simulink model "microwave_class_updated"  (Simulink 8.5)
settings: Solver=FixedStepDiscrete  StartTime=0.0  StopTime=inf  MaxStep=1  RelTol=1e-3
libraries: microwave_class_defs x36, sldvlib x21, powerlib_meascontrol x13, simulink x9
settings Model: Creator=spmiller  LastModifiedBy=Elaheh
settings DataIOCC: SaveFormat=Structure
settings OptimizationCC: InitFltsAndDblsToZero=on
settings DebuggingCC: SaveWithParameterizedLinksMsg=none  SignalResolutionControl=TryResolveAllWithWarning  SolverPrmCheckMsg=warning  MultiTaskDSMMsg=warning  MultiTaskCondExecSysMsg=none  FcnCallInpInsideContextMsg=UseLocalSettings
settings SFSimCC: SimParseCustomCode=off
settings GRTTargetCC: TargetFcnLib=ansi_tfl_tmw.mat

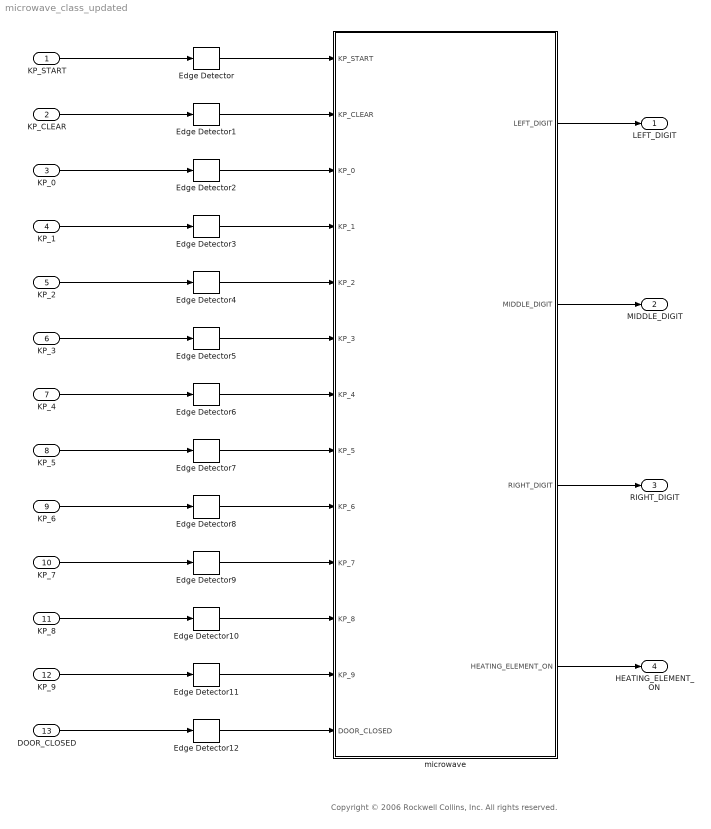
== system microwave_class_updated ==
  note: Copyright © 2006 Rockwell Collins, Inc. All rights reserved.
  KP_START : Inport  OutDataTypeStr=boolean
  KP_CLEAR : Inport  Port=2  OutDataTypeStr=boolean
  KP_0 : Inport  Port=3  OutDataTypeStr=boolean
  KP_1 : Inport  Port=4  OutDataTypeStr=boolean
  KP_2 : Inport  Port=5  OutDataTypeStr=boolean
  KP_3 : Inport  Port=6  OutDataTypeStr=boolean
  KP_4 : Inport  Port=7  OutDataTypeStr=boolean
  KP_5 : Inport  Port=8  OutDataTypeStr=boolean
  KP_6 : Inport  Port=9  OutDataTypeStr=boolean
  KP_7 : Inport  Port=10  OutDataTypeStr=boolean
  KP_8 : Inport  Port=11  OutDataTypeStr=boolean
  KP_9 : Inport  Port=12  OutDataTypeStr=boolean
  DOOR_CLOSED : Inport  Port=13  OutDataTypeStr=boolean
  Edge Detector{,1..12} (13 alike) : powerlib_meascontrol/Logic/Edge Detector  model=Rising  ic=0  Ts=0
  microwave : Subsystem
  LEFT_DIGIT : Outport  OutDataTypeStr=int8
  MIDDLE_DIGIT : Outport  Port=2  OutDataTypeStr=int8
  RIGHT_DIGIT : Outport  Port=3  OutDataTypeStr=int8
  HEATING_ELEMENT_ON : Outport  Port=4  OutDataTypeStr=boolean
  wires:
  KP_START/1 -> Edge Detector/1
  microwave/2(MIDDLE_DIGIT) -> MIDDLE_DIGIT/1
  microwave/3(RIGHT_DIGIT) -> RIGHT_DIGIT/1
  microwave/4(HEATING_ELEMENT_ON) -> HEATING_ELEMENT_ON/1
  microwave/1(LEFT_DIGIT) -> LEFT_DIGIT/1
  KP_3/1 -> Edge Detector5/1
  KP_4/1 -> Edge Detector6/1
  KP_6/1 -> Edge Detector8/1
  KP_7/1 -> Edge Detector9/1
  KP_9/1 -> Edge Detector11/1
  DOOR_CLOSED/1 -> Edge Detector12/1
  Edge Detector/1 -> microwave/1(KP_START)
  KP_CLEAR/1 -> Edge Detector1/1
  Edge Detector1/1 -> microwave/2(KP_CLEAR)
  KP_0/1 -> Edge Detector2/1
  Edge Detector2/1 -> microwave/3(KP_0)
  KP_1/1 -> Edge Detector3/1
  Edge Detector3/1 -> microwave/4(KP_1)
  KP_2/1 -> Edge Detector4/1
  Edge Detector4/1 -> microwave/5(KP_2)
  Edge Detector5/1 -> microwave/6(KP_3)
  Edge Detector6/1 -> microwave/7(KP_4)
  Edge Detector7/1 -> microwave/8(KP_5)
  KP_5/1 -> Edge Detector7/1
  Edge Detector8/1 -> microwave/9(KP_6)
  Edge Detector9/1 -> microwave/10(KP_7)
  Edge Detector10/1 -> microwave/11(KP_8)
  KP_8/1 -> Edge Detector10/1
  Edge Detector11/1 -> microwave/12(KP_9)
  Edge Detector12/1 -> microwave/13(DOOR_CLOSED)

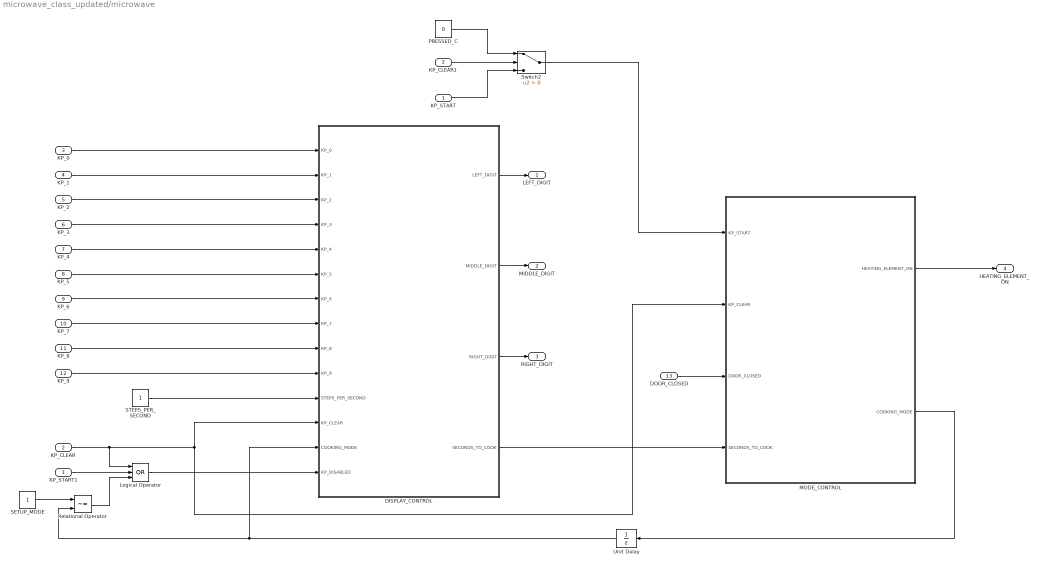
== system microwave_class_updated/microwave ==
  KP_START : Inport  OutDataTypeStr=boolean
  KP_CLEAR : Inport  Port=2  OutDataTypeStr=boolean
  KP_0 : Inport  Port=3  OutDataTypeStr=boolean
  KP_1 : Inport  Port=4  OutDataTypeStr=boolean
  KP_2 : Inport  Port=5  OutDataTypeStr=boolean
  KP_3 : Inport  Port=6  OutDataTypeStr=boolean
  KP_4 : Inport  Port=7  OutDataTypeStr=boolean
  KP_5 : Inport  Port=8  OutDataTypeStr=boolean
  KP_6 : Inport  Port=9  OutDataTypeStr=boolean
  KP_7 : Inport  Port=10  OutDataTypeStr=boolean
  KP_8 : Inport  Port=11  OutDataTypeStr=boolean
  KP_9 : Inport  Port=12  OutDataTypeStr=boolean
  DOOR_CLOSED : Inport  Port=13  OutDataTypeStr=boolean
  DISPLAY_CONTROL : Subsystem
  KP_CLEAR1 : InportShadow  Port=2  OutDataTypeStr=boolean
  KP_START1 : InportShadow  OutDataTypeStr=boolean
  Logical Operator : Logic  Operator=OR  Inputs=3  AllPortsSameDT=off  OutDataTypeStr=boolean
  MODE_CONTROL : Subsystem
  PRESSED_C : Constant  Value=0  OutDataTypeStr=boolean
  Relational Operator : RelationalOperator  Operator=~=  OutDataTypeStr=boolean
  SETUP_MODE : Constant  OutDataTypeStr=int8
  STEPS_PER_SECOND : Constant  OutDataTypeStr=int8
  Switch2 : Switch  Criteria=u2 > Threshold
  Unit Delay : UnitDelay  SampleTime=-1
  LEFT_DIGIT : Outport  OutDataTypeStr=int8
  MIDDLE_DIGIT : Outport  Port=2  OutDataTypeStr=int8
  RIGHT_DIGIT : Outport  Port=3  OutDataTypeStr=int8
  HEATING_ELEMENT_ON : Outport  Port=4  OutDataTypeStr=boolean
  wires:
  KP_CLEAR/1 -> Logical Operator/1, DISPLAY_CONTROL/12(KP_CLEAR), MODE_CONTROL/2(KP_CLEAR)
  DISPLAY_CONTROL/4(SECONDS_TO_COOK) -> MODE_CONTROL/4(SECONDS_TO_COOK)
  MODE_CONTROL/2(COOKING_MODE) -> Unit Delay/1
  Unit Delay/1 -> Relational Operator/2, DISPLAY_CONTROL/13(COOKING_MODE)
  DOOR_CLOSED/1 -> MODE_CONTROL/3(DOOR_CLOSED)
  DISPLAY_CONTROL/3(RIGHT_DIGIT) -> RIGHT_DIGIT/1
  DISPLAY_CONTROL/2(MIDDLE_DIGIT) -> MIDDLE_DIGIT/1
  DISPLAY_CONTROL/1(LEFT_DIGIT) -> LEFT_DIGIT/1
  MODE_CONTROL/1(HEATING_ELEMENT_ON) -> HEATING_ELEMENT_ON/1
  STEPS_PER_SECOND/1 -> DISPLAY_CONTROL/11(STEPS_PER_SECOND)
  KP_CLEAR1/1 -> Switch2/2
  PRESSED_C/1 -> Switch2/1
  KP_START/1 -> Switch2/3
  KP_1/1 -> DISPLAY_CONTROL/2(KP_1)
  KP_3/1 -> DISPLAY_CONTROL/4(KP_3)
  KP_4/1 -> DISPLAY_CONTROL/5(KP_4)
  KP_5/1 -> DISPLAY_CONTROL/6(KP_5)
  KP_6/1 -> DISPLAY_CONTROL/7(KP_6)
  KP_7/1 -> DISPLAY_CONTROL/8(KP_7)
  KP_2/1 -> DISPLAY_CONTROL/3(KP_2)
  KP_8/1 -> DISPLAY_CONTROL/9(KP_8)
  KP_9/1 -> DISPLAY_CONTROL/10(KP_9)
  KP_0/1 -> DISPLAY_CONTROL/1(KP_0)
  KP_START1/1 -> Logical Operator/2
  Logical Operator/1 -> DISPLAY_CONTROL/14(KP_DISABLED)
  Relational Operator/1 -> Logical Operator/3
  SETUP_MODE/1 -> Relational Operator/1
  Switch2/1 -> MODE_CONTROL/1(KP_START)

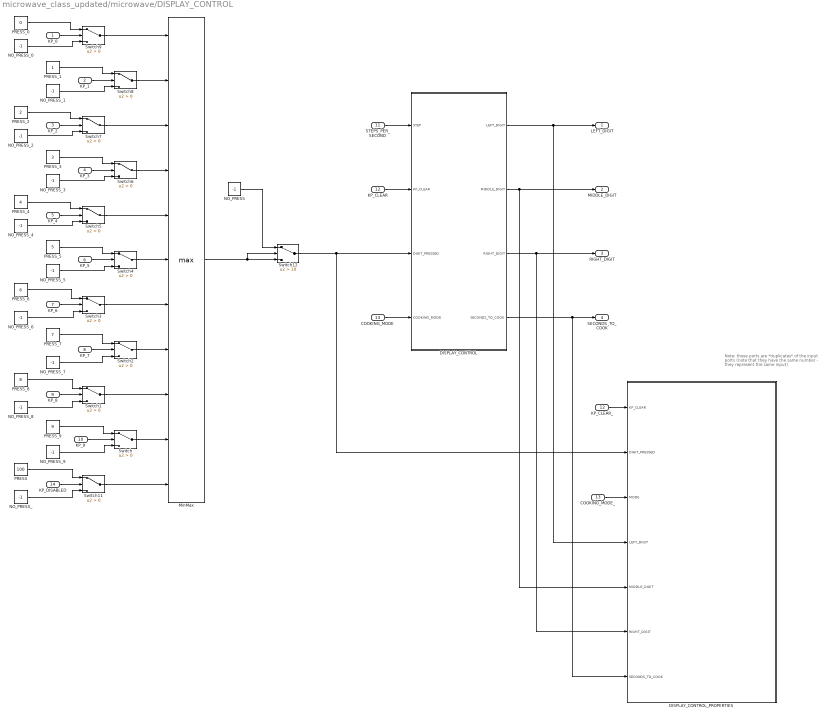
== system microwave_class_updated/microwave/DISPLAY_CONTROL ==
  note: Note: these ports are *duplicates* of the
      | input ports (note that they have the same
      | number - they represent the same input)
  KP_0 : Inport
  KP_1 : Inport  Port=2
  KP_2 : Inport  Port=3
  KP_3 : Inport  Port=4
  KP_4 : Inport  Port=5
  KP_5 : Inport  Port=6
  KP_6 : Inport  Port=7
  KP_7 : Inport  Port=8
  KP_8 : Inport  Port=9
  KP_9 : Inport  Port=10
  STEPS_PER_SECOND : Inport  Port=11  OutDataTypeStr=int8
  KP_CLEAR : Inport  Port=12
  COOKING_MODE : Inport  Port=13  OutDataTypeStr=uint8
  KP_DISABLED : Inport  Port=14
  COOKING_MODE_ : InportShadow  Port=13  OutDataTypeStr=uint8
  DISPLAY_CONTROL : Stateflow chart  TreatAsAtomicUnit=on
  DISPLAY_CONTROL_PROPERTIES : Subsystem
  KP_CLEAR_ : InportShadow  Port=12
  MinMax : MinMax  Function=max  Inputs=11
  NO_PRESS : Constant  Value=-1  OutDataTypeStr=int8
  NO_PRESS_{,0..9} (11 alike) : Constant  Value=-1  OutDataTypeStr=int8
  PRESS : Constant  Value=100  OutDataTypeStr=int8
  PRESS_0 : Constant  Value=0  OutDataTypeStr=int8
  PRESS_1 : Constant  OutDataTypeStr=int8
  PRESS_2 : Constant  Value=2  OutDataTypeStr=int8
  PRESS_3 : Constant  Value=3  OutDataTypeStr=int8
  PRESS_4 : Constant  Value=4  OutDataTypeStr=int8
  PRESS_5 : Constant  Value=5  OutDataTypeStr=int8
  PRESS_6 : Constant  Value=6  OutDataTypeStr=int8
  PRESS_7 : Constant  Value=7  OutDataTypeStr=int8
  PRESS_8 : Constant  Value=8  OutDataTypeStr=int8
  PRESS_9 : Constant  Value=9  OutDataTypeStr=int8
  Switch{,1..9,11} (11 alike) : Switch  Criteria=u2 > Threshold
  Switch12 : Switch  Criteria=u2 > Threshold  Threshold=10
  LEFT_DIGIT : Outport  OutDataTypeStr=int8
  MIDDLE_DIGIT : Outport  Port=2  OutDataTypeStr=int8
  RIGHT_DIGIT : Outport  Port=3  OutDataTypeStr=int8
  SECONDS_TO_COOK : Outport  Port=4  OutDataTypeStr=int8
  wires:
  STEPS_PER_SECOND/1 -> DISPLAY_CONTROL/1(STEP)
  DISPLAY_CONTROL/1(LEFT_DIGIT) -> DISPLAY_CONTROL_PROPERTIES/4(LEFT_DIGIT), LEFT_DIGIT/1
  DISPLAY_CONTROL/3(RIGHT_DIGIT) -> RIGHT_DIGIT/1, DISPLAY_CONTROL_PROPERTIES/6(RIGHT_DIGIT)
  DISPLAY_CONTROL/2(MIDDLE_DIGIT) -> DISPLAY_CONTROL_PROPERTIES/5(MIDDLE_DIGIT), MIDDLE_DIGIT/1
  KP_CLEAR/1 -> DISPLAY_CONTROL/2(KP_CLEAR)
  NO_PRESS_9/1 -> Switch/3
  KP_9/1 -> Switch/2
  PRESS_9/1 -> Switch/1
  PRESS_8/1 -> Switch1/1
  NO_PRESS_8/1 -> Switch1/3
  KP_8/1 -> Switch1/2
  KP_7/1 -> Switch2/2
  PRESS_7/1 -> Switch2/1
  NO_PRESS_7/1 -> Switch2/3
  KP_6/1 -> Switch3/2
  PRESS_6/1 -> Switch3/1
  NO_PRESS_6/1 -> Switch3/3
  KP_5/1 -> Switch4/2
  PRESS_5/1 -> Switch4/1
  NO_PRESS_5/1 -> Switch4/3
  PRESS_4/1 -> Switch5/1
  NO_PRESS_4/1 -> Switch5/3
  KP_4/1 -> Switch5/2
  KP_3/1 -> Switch6/2
  PRESS_3/1 -> Switch6/1
  NO_PRESS_3/1 -> Switch6/3
  PRESS_2/1 -> Switch7/1
  NO_PRESS_2/1 -> Switch7/3
  KP_2/1 -> Switch7/2
  KP_1/1 -> Switch8/2
  PRESS_1/1 -> Switch8/1
  NO_PRESS_1/1 -> Switch8/3
  PRESS_0/1 -> Switch9/1
  NO_PRESS_0/1 -> Switch9/3
  KP_0/1 -> Switch9/2
  Switch2/1 -> MinMax/8
  Switch1/1 -> MinMax/9
  Switch/1 -> MinMax/10
  COOKING_MODE_/1 -> DISPLAY_CONTROL_PROPERTIES/3(MODE)
  KP_CLEAR_/1 -> DISPLAY_CONTROL_PROPERTIES/1(KP_CLEAR)
  COOKING_MODE/1 -> DISPLAY_CONTROL/4(COOKING_MODE)
  DISPLAY_CONTROL/4(SECONDS_TO_COOK) -> DISPLAY_CONTROL_PROPERTIES/7(SECONDS_TO_COOK), SECONDS_TO_COOK/1
  Switch3/1 -> MinMax/7
  Switch4/1 -> MinMax/6
  Switch5/1 -> MinMax/5
  Switch6/1 -> MinMax/4
  Switch7/1 -> MinMax/3
  Switch8/1 -> MinMax/2
  Switch9/1 -> MinMax/1
  Switch12/1 -> DISPLAY_CONTROL_PROPERTIES/2(DIGIT_PRESSED), DISPLAY_CONTROL/3(DIGIT_PRESSED)
  NO_PRESS/1 -> Switch12/1
  PRESS/1 -> Switch11/1
  NO_PRESS_/1 -> Switch11/3
  KP_DISABLED/1 -> Switch11/2
  Switch11/1 -> MinMax/11
  MinMax/1 -> Switch12/2, Switch12/3

== system microwave_class_updated/microwave/MODE_CONTROL ==
  KP_START : Inport  OutDataTypeStr=boolean
  KP_CLEAR : Inport  Port=2  OutDataTypeStr=boolean
  DOOR_CLOSED : Inport  Port=3  OutDataTypeStr=boolean
  SECONDS_TO_COOK : Inport  Port=4
  MODE_CONTROL : Stateflow chart  TreatAsAtomicUnit=on
  MODE_CONTROL_PROPERTIES : Subsystem
  HEATING_ELEMENT_ON : Outport
  COOKING_MODE : Outport  Port=2
  wires:
  KP_START/1 -> MODE_CONTROL_PROPERTIES/1(KP_START), MODE_CONTROL/1(KP_START)
  KP_CLEAR/1 -> MODE_CONTROL_PROPERTIES/2(KP_CLEAR), MODE_CONTROL/2(KP_CLEAR)
  DOOR_CLOSED/1 -> MODE_CONTROL_PROPERTIES/3(DOOR_CLOSED), MODE_CONTROL/3(DOOR_CLOSED)
  SECONDS_TO_COOK/1 -> MODE_CONTROL_PROPERTIES/4(SECONDS_TO_COOK), MODE_CONTROL/4(SECONDS_TO_COOK)
  MODE_CONTROL/1(COOKING_MODE) -> MODE_CONTROL_PROPERTIES/5(COOKING_MODE), COOKING_MODE/1
  MODE_CONTROL/2(HEATING_ELEMENT_ON) -> MODE_CONTROL_PROPERTIES/6(HEATING_ELEMENT_ON), HEATING_ELEMENT_ON/1

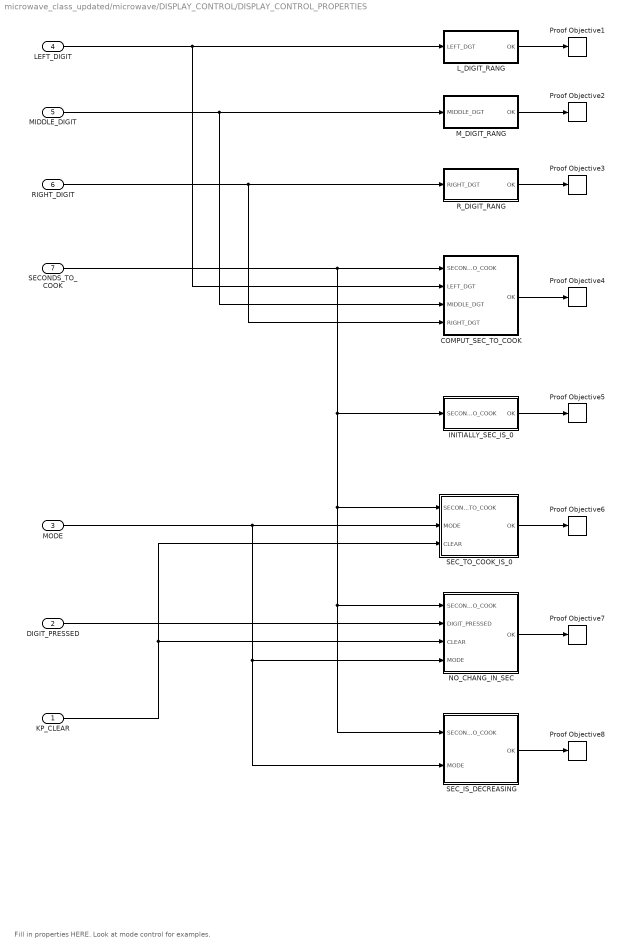
== system microwave_class_updated/microwave/DISPLAY_CONTROL/DISPLAY_CONTROL_PROPERTIES ==
  note: Fill in properties HERE. Look at mode control for examples.
  KP_CLEAR : Inport  OutDataTypeStr=boolean
  DIGIT_PRESSED : Inport  Port=2  OutDataTypeStr=int8
  MODE : Inport  Port=3  OutDataTypeStr=uint8
  LEFT_DIGIT : Inport  Port=4  OutDataTypeStr=int8
  MIDDLE_DIGIT : Inport  Port=5  OutDataTypeStr=int8
  RIGHT_DIGIT : Inport  Port=6  OutDataTypeStr=int8
  SECONDS_TO_COOK : Inport  Port=7
  COMPUT_SEC_TO_COOK : Subsystem
  INITIALLY_SEC_IS_0 : Subsystem
  L_DIGIT_RANG : Subsystem
  M_DIGIT_RANG : Subsystem
  NO_CHANG_IN_SEC : Subsystem
  Proof Objective{1..8} (8 alike) : sldvlib/Objectives and Constraints/Proof Objective  enabled=on  customAVTBlockType=Proof Objective  intervals=true  dispValues=on  outEnabled=on  enableStopSim=off
      settings: AttributesFormatString=%<intervals>
  R_DIGIT_RANG : Subsystem
  SEC_IS_DECREASING : Subsystem
  SEC_TO_COOK_IS_0 : Subsystem
  wires:
  L_DIGIT_RANG/1(OK) -> Proof Objective1/1
  M_DIGIT_RANG/1(OK) -> Proof Objective2/1
  R_DIGIT_RANG/1(OK) -> Proof Objective3/1
  COMPUT_SEC_TO_COOK/1(OK) -> Proof Objective4/1
  INITIALLY_SEC_IS_0/1(OK) -> Proof Objective5/1
  SEC_TO_COOK_IS_0/1(OK) -> Proof Objective6/1
  NO_CHANG_IN_SEC/1(OK) -> Proof Objective7/1
  SEC_IS_DECREASING/1(OK) -> Proof Objective8/1
  MODE/1 -> SEC_IS_DECREASING/2(MODE), NO_CHANG_IN_SEC/4(MODE), SEC_TO_COOK_IS_0/2(MODE)
  LEFT_DIGIT/1 -> COMPUT_SEC_TO_COOK/2(LEFT_DGT), L_DIGIT_RANG/1(LEFT_DGT)
  MIDDLE_DIGIT/1 -> COMPUT_SEC_TO_COOK/3(MIDDLE_DGT), M_DIGIT_RANG/1(MIDDLE_DGT)
  SECONDS_TO_COOK/1 -> SEC_IS_DECREASING/1(SECONDS_TO_COOK), NO_CHANG_IN_SEC/1(SECONDS_TO_COOK), SEC_TO_COOK_IS_0/1(SECONDS_TO_COOK), INITIALLY_SEC_IS_0/1(SECONDS_TO_COOK), COMPUT_SEC_TO_COOK/1(SECONDS_TO_COOK)
  DIGIT_PRESSED/1 -> NO_CHANG_IN_SEC/2(DIGIT_PRESSED)
  KP_CLEAR/1 -> SEC_TO_COOK_IS_0/3(CLEAR), NO_CHANG_IN_SEC/3(CLEAR)
  RIGHT_DIGIT/1 -> COMPUT_SEC_TO_COOK/4(RIGHT_DGT), R_DIGIT_RANG/1(RIGHT_DGT)

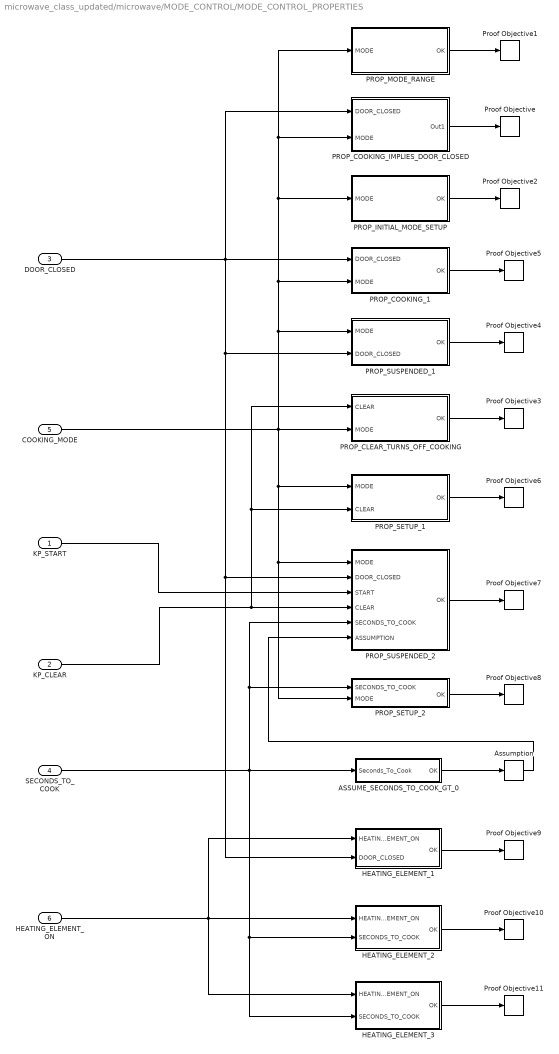
== system microwave_class_updated/microwave/MODE_CONTROL/MODE_CONTROL_PROPERTIES ==
  KP_START : Inport  OutDataTypeStr=boolean
  KP_CLEAR : Inport  Port=2  OutDataTypeStr=boolean
  DOOR_CLOSED : Inport  Port=3  OutDataTypeStr=boolean
  SECONDS_TO_COOK : Inport  Port=4
  COOKING_MODE : Inport  Port=5  OutDataTypeStr=uint8
  HEATING_ELEMENT_ON : Inport  Port=6  OutDataTypeStr=boolean
  ASSUME_SECONDS_TO_COOK_GT_0 : Subsystem
  Assumption : sldvlib/Objectives and Constraints/Assumption  enabled=on  customAVTBlockType=Assumption  intervals=true  initial=off  dispValues=on  outEnabled=on
      settings: AttributesFormatString=%<intervals>
  HEATING_ELEMENT_1 : Subsystem
  HEATING_ELEMENT_2 : Subsystem
  HEATING_ELEMENT_3 : Subsystem
  PROP_CLEAR_TURNS_OFF_COOKING : Subsystem
  PROP_COOKING_1 : Subsystem
  PROP_COOKING_IMPLIES_DOOR_CLOSED : Subsystem
  PROP_INITIAL_MODE_SETUP : Subsystem
  PROP_MODE_RANGE : Subsystem
  PROP_SETUP_1 : Subsystem
  PROP_SETUP_2 : Subsystem
  PROP_SUSPENDED_1 : Subsystem
  PROP_SUSPENDED_2 : Subsystem
  Proof Objective{,1..11} (12 alike) : sldvlib/Objectives and Constraints/Proof Objective  enabled=on  customAVTBlockType=Proof Objective  intervals=true  dispValues=on  outEnabled=on  enableStopSim=off
      settings: AttributesFormatString=%<intervals>
  wires:
  COOKING_MODE/1 -> PROP_SUSPENDED_1/1(MODE), PROP_INITIAL_MODE_SETUP/1(MODE), PROP_MODE_RANGE/1(MODE), PROP_COOKING_IMPLIES_DOOR_CLOSED/2(MODE), PROP_COOKING_1/2(MODE), PROP_SETUP_2/2(MODE), PROP_SUSPENDED_2/1(MODE), PROP_SETUP_1/1(MODE), PROP_CLEAR_TURNS_OFF_COOKING/2(MODE)
  PROP_COOKING_IMPLIES_DOOR_CLOSED/1(Out1) -> Proof Objective/1
  PROP_CLEAR_TURNS_OFF_COOKING/1(OK) -> Proof Objective3/1
  ASSUME_SECONDS_TO_COOK_GT_0/1(OK) -> Assumption/1
  PROP_MODE_RANGE/1(OK) -> Proof Objective1/1
  PROP_INITIAL_MODE_SETUP/1(OK) -> Proof Objective2/1
  PROP_SUSPENDED_1/1(OK) -> Proof Objective4/1
  PROP_COOKING_1/1(OK) -> Proof Objective5/1
  PROP_SETUP_1/1(OK) -> Proof Objective6/1
  PROP_SUSPENDED_2/1(OK) -> Proof Objective7/1
  PROP_SETUP_2/1(OK) -> Proof Objective8/1
  KP_CLEAR/1 -> PROP_CLEAR_TURNS_OFF_COOKING/1(CLEAR), PROP_SETUP_1/2(CLEAR), PROP_SUSPENDED_2/4(CLEAR)
  DOOR_CLOSED/1 -> PROP_COOKING_IMPLIES_DOOR_CLOSED/1(DOOR_CLOSED), HEATING_ELEMENT_1/2(DOOR_CLOSED), PROP_SUSPENDED_2/2(DOOR_CLOSED), PROP_SUSPENDED_1/2(DOOR_CLOSED), PROP_COOKING_1/1(DOOR_CLOSED)
  KP_START/1 -> PROP_SUSPENDED_2/3(START)
  SECONDS_TO_COOK/1 -> HEATING_ELEMENT_2/2(SECONDS_TO_COOK), HEATING_ELEMENT_3/2(SECONDS_TO_COOK), PROP_SUSPENDED_2/5(SECONDS_TO_COOK), PROP_SETUP_2/1(SECONDS_TO_COOK), ASSUME_SECONDS_TO_COOK_GT_0/1(Seconds_To_Cook)
  HEATING_ELEMENT_1/1(OK) -> Proof Objective9/1
  HEATING_ELEMENT_2/1(OK) -> Proof Objective10/1
  HEATING_ELEMENT_3/1(OK) -> Proof Objective11/1
  HEATING_ELEMENT_ON/1 -> HEATING_ELEMENT_1/1(HEATING_ELEMENT_ON), HEATING_ELEMENT_3/1(HEATING_ELEMENT_ON), HEATING_ELEMENT_2/1(HEATING_ELEMENT_ON)
  Assumption/1 -> PROP_SUSPENDED_2/6(ASSUMPTION)

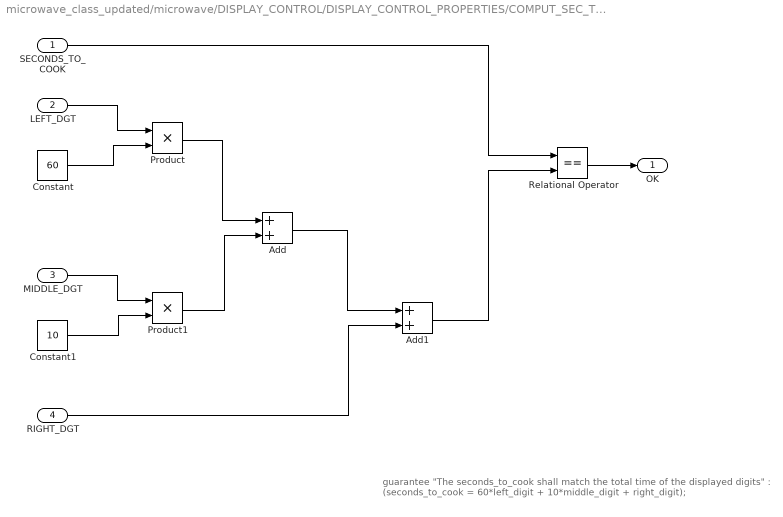
== system microwave_class_updated/microwave/DISPLAY_CONTROL/DISPLAY_CONTROL_PROPERTIES/COMPUT_SEC_TO_COOK ==
  note: guarantee "The seconds_to_cook shall match the total time of the displayed digits" :
      | 			(seconds_to_cook = 60*left_digit + 10*middle_digit + right_digit);
  SECONDS_TO_COOK : Inport
  LEFT_DGT : Inport  Port=2
  MIDDLE_DGT : Inport  Port=3
  RIGHT_DGT : Inport  Port=4
  Add : Sum
  Add1 : Sum
  Constant : Constant  Value=60
  Constant1 : Constant  Value=10
  Product : Product
  Product1 : Product
  Relational Operator : RelationalOperator  Operator===  OutDataTypeStr=boolean
  OK : Outport
  wires:
  SECONDS_TO_COOK/1 -> Relational Operator/1
  Relational Operator/1 -> OK/1
  LEFT_DGT/1 -> Product/1
  Constant/1 -> Product/2
  Product/1 -> Add/1
  MIDDLE_DGT/1 -> Product1/1
  Constant1/1 -> Product1/2
  Product1/1 -> Add/2
  RIGHT_DGT/1 -> Add1/2
  Add/1 -> Add1/1
  Add1/1 -> Relational Operator/2

== system microwave_class_updated/microwave/DISPLAY_CONTROL/DISPLAY_CONTROL_PROPERTIES/INITIALLY_SEC_IS_0 ==
  note: guarantee "Seconds to cook shall be initially zero" :
      | 			std.Initially(seconds_to_cook = 0);
  SECONDS_TO_COOK : Inport
  Constant : Constant  Value=0
  Relational Operator : RelationalOperator  Operator===  OutDataTypeStr=boolean
  initially_true : microwave_class_defs/initially_true
  OK : Outport
  wires:
  SECONDS_TO_COOK/1 -> Relational Operator/1
  Constant/1 -> Relational Operator/2
  Relational Operator/1 -> initially_true/1
  initially_true/1 -> OK/1

== system microwave_class_updated/microwave/DISPLAY_CONTROL/DISPLAY_CONTROL_PROPERTIES/L_DIGIT_RANG ==
  note: guarantee "left_digit range shall be [0..9]" :
      | 			(left_digit >= 0 and left_digit <= 9);
  LEFT_DGT : Inport
  Compare To Zero : simulink/Logic and Bit Operations/Compare To Zero  relop=>=  OutDataTypeStr=boolean
  Constant1 : Constant  Value=9
  Logical Operator : Logic  AllPortsSameDT=off  OutDataTypeStr=boolean
  Relational Operator : RelationalOperator  Operator=<=  OutDataTypeStr=boolean
  OK : Outport
  wires:
  LEFT_DGT/1 -> Compare To Zero/1, Relational Operator/1
  Constant1/1 -> Relational Operator/2
  Compare To Zero/1 -> Logical Operator/1
  Relational Operator/1 -> Logical Operator/2
  Logical Operator/1 -> OK/1

== system microwave_class_updated/microwave/DISPLAY_CONTROL/DISPLAY_CONTROL_PROPERTIES/M_DIGIT_RANG ==
  note: guarantee "middle_digit range shall be [0..9]" :
      | 			(middle_digit >= 0 and middle_digit <= 9);
  MIDDLE_DGT : Inport
  Compare To Zero : simulink/Logic and Bit Operations/Compare To Zero  relop=>=  OutDataTypeStr=boolean
  Constant1 : Constant  Value=9
  Logical Operator : Logic  AllPortsSameDT=off  OutDataTypeStr=boolean
  Relational Operator : RelationalOperator  Operator=<=  OutDataTypeStr=boolean
  OK : Outport
  wires:
  MIDDLE_DGT/1 -> Compare To Zero/1, Relational Operator/1
  Constant1/1 -> Relational Operator/2
  Compare To Zero/1 -> Logical Operator/1
  Relational Operator/1 -> Logical Operator/2
  Logical Operator/1 -> OK/1

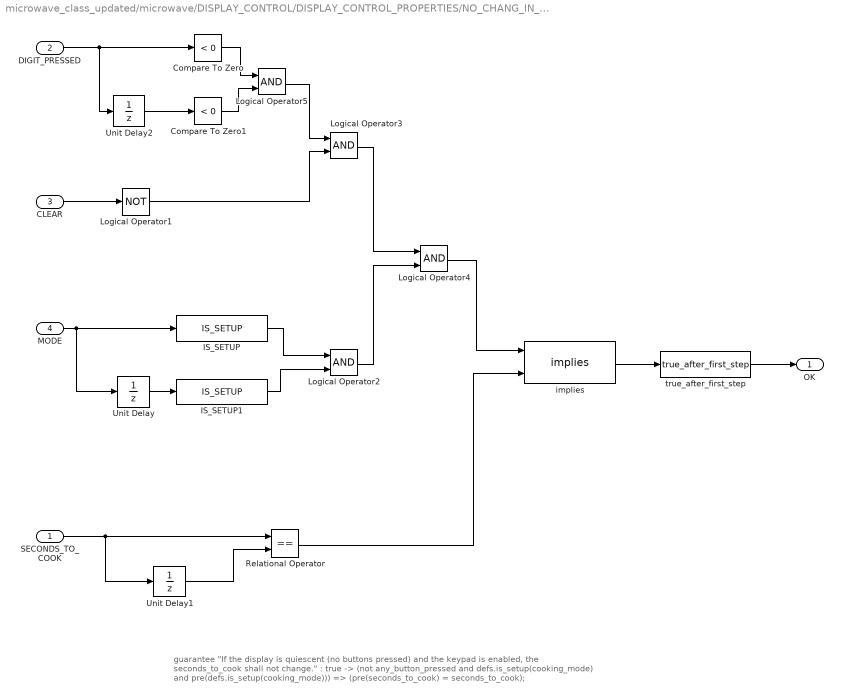
== system microwave_class_updated/microwave/DISPLAY_CONTROL/DISPLAY_CONTROL_PROPERTIES/NO_CHANG_IN_SEC ==
  note: guarantee "If the display is quiescent (no buttons pressed) and the keypad is enabled, the seconds_to_cook shall not change." :
      | 			true -> (not any_button_pressed and defs.is_setup(cooking_mode) and pre(defs.is_setup(cooking_mode))) => (pre(seconds_to_cook) = seconds_to_cook);
  SECONDS_TO_COOK : Inport
  DIGIT_PRESSED : Inport  Port=2
  CLEAR : Inport  Port=3
  MODE : Inport  Port=4
  Compare To Zero : simulink/Logic and Bit Operations/Compare To Zero  relop=<  OutDataTypeStr=boolean
  Compare To Zero1 : simulink/Logic and Bit Operations/Compare To Zero  relop=<  OutDataTypeStr=boolean
  IS_SETUP : microwave_class_defs/IS_SETUP
  IS_SETUP1 : microwave_class_defs/IS_SETUP
  Logical Operator1 : Logic  Operator=NOT  AllPortsSameDT=off  OutDataTypeStr=boolean
  Logical Operator{2..5} (4 alike) : Logic  AllPortsSameDT=off  OutDataTypeStr=boolean
  Relational Operator : RelationalOperator  Operator===  OutDataTypeStr=boolean
  Unit Delay : UnitDelay  SampleTime=-1
  Unit Delay1 : UnitDelay  SampleTime=-1
  Unit Delay2 : UnitDelay  SampleTime=-1
  implies : microwave_class_defs/implies
  true_after_first_step : microwave_class_defs/true_after_first_step
  OK : Outport
  wires:
  Logical Operator1/1 -> Logical Operator3/2
  Logical Operator3/1 -> Logical Operator4/1
  Relational Operator/1 -> implies/2
  implies/1 -> true_after_first_step/1
  true_after_first_step/1 -> OK/1
  CLEAR/1 -> Logical Operator1/1
  MODE/1 -> Unit Delay/1, IS_SETUP/1
  Unit Delay/1 -> IS_SETUP1/1
  IS_SETUP1/1 -> Logical Operator2/2
  IS_SETUP/1 -> Logical Operator2/1
  Logical Operator2/1 -> Logical Operator4/2
  Logical Operator4/1 -> implies/1
  SECONDS_TO_COOK/1 -> Unit Delay1/1, Relational Operator/1
  Unit Delay1/1 -> Relational Operator/2
  DIGIT_PRESSED/1 -> Unit Delay2/1, Compare To Zero/1
  Unit Delay2/1 -> Compare To Zero1/1
  Compare To Zero/1 -> Logical Operator5/1
  Compare To Zero1/1 -> Logical Operator5/2
  Logical Operator5/1 -> Logical Operator3/1

== system microwave_class_updated/microwave/DISPLAY_CONTROL/DISPLAY_CONTROL_PROPERTIES/R_DIGIT_RANG ==
  note: guarantee "right_digit range shall be [0..9]" :
      | 			(right_digit >= 0 and right_digit <= 9);
  RIGHT_DGT : Inport
  Compare To Zero : simulink/Logic and Bit Operations/Compare To Zero  relop=>=  OutDataTypeStr=boolean
  Constant1 : Constant  Value=9
  Logical Operator : Logic  AllPortsSameDT=off  OutDataTypeStr=boolean
  Relational Operator : RelationalOperator  Operator=<=  OutDataTypeStr=boolean
  OK : Outport
  wires:
  RIGHT_DGT/1 -> Compare To Zero/1, Relational Operator/1
  Constant1/1 -> Relational Operator/2
  Compare To Zero/1 -> Logical Operator/1
  Relational Operator/1 -> Logical Operator/2
  Logical Operator/1 -> OK/1

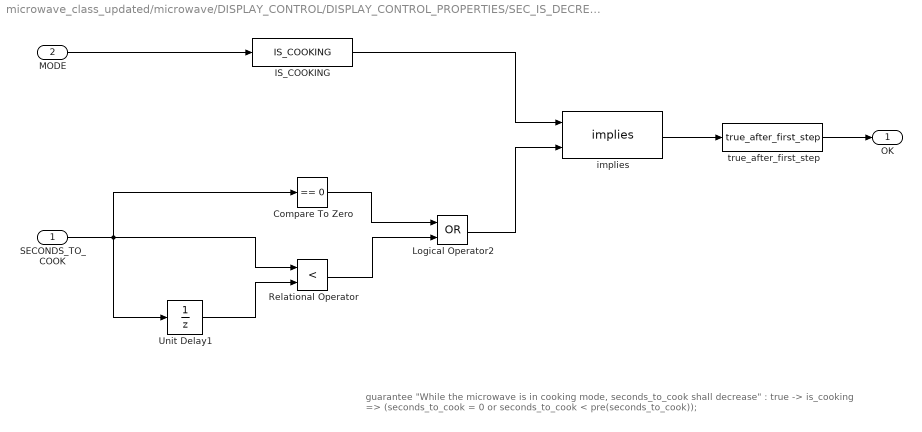
== system microwave_class_updated/microwave/DISPLAY_CONTROL/DISPLAY_CONTROL_PROPERTIES/SEC_IS_DECREASING ==
  note: guarantee "While the microwave is in cooking mode, seconds_to_cook shall decrease" :
      | 			true -> is_cooking => (seconds_to_cook = 0 or seconds_to_cook < pre(seconds_to_cook));
  SECONDS_TO_COOK : Inport
  MODE : Inport  Port=2
  Compare To Zero : simulink/Logic and Bit Operations/Compare To Zero  relop===  OutDataTypeStr=boolean
  IS_COOKING : microwave_class_defs/IS_COOKING
  Logical Operator2 : Logic  Operator=OR  AllPortsSameDT=off  OutDataTypeStr=boolean
  Relational Operator : RelationalOperator  Operator=<  OutDataTypeStr=boolean
  Unit Delay1 : UnitDelay  SampleTime=-1
  implies : microwave_class_defs/implies
  true_after_first_step : microwave_class_defs/true_after_first_step
  OK : Outport
  wires:
  Relational Operator/1 -> Logical Operator2/2
  implies/1 -> true_after_first_step/1
  true_after_first_step/1 -> OK/1
  MODE/1 -> IS_COOKING/1
  Logical Operator2/1 -> implies/2
  SECONDS_TO_COOK/1 -> Unit Delay1/1, Relational Operator/1, Compare To Zero/1
  Unit Delay1/1 -> Relational Operator/2
  Compare To Zero/1 -> Logical Operator2/1
  IS_COOKING/1 -> implies/1

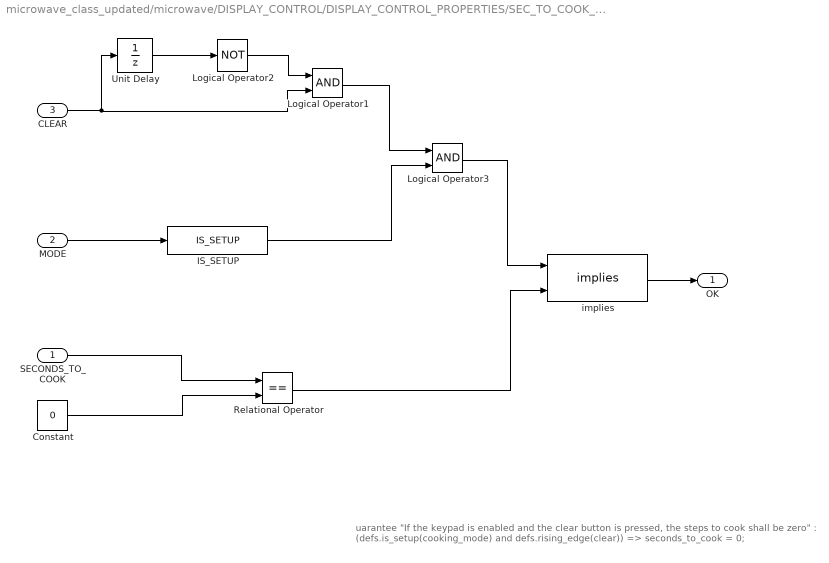
== system microwave_class_updated/microwave/DISPLAY_CONTROL/DISPLAY_CONTROL_PROPERTIES/SEC_TO_COOK_IS_0 ==
  note: uarantee "If the keypad is enabled and the clear button is pressed, the steps to cook shall be zero" :
      | 			(defs.is_setup(cooking_mode) and  defs.rising_edge(clear)) => seconds_to_cook = 0;
  SECONDS_TO_COOK : Inport
  MODE : Inport  Port=2
  CLEAR : Inport  Port=3
  Constant : Constant  Value=0
  IS_SETUP : microwave_class_defs/IS_SETUP
  Logical Operator1 : Logic  AllPortsSameDT=off  OutDataTypeStr=boolean
  Logical Operator2 : Logic  Operator=NOT  AllPortsSameDT=off  OutDataTypeStr=boolean
  Logical Operator3 : Logic  AllPortsSameDT=off  OutDataTypeStr=boolean
  Relational Operator : RelationalOperator  Operator===  OutDataTypeStr=boolean
  Unit Delay : UnitDelay  SampleTime=-1
  implies : microwave_class_defs/implies
  OK : Outport
  wires:
  SECONDS_TO_COOK/1 -> Relational Operator/1
  Constant/1 -> Relational Operator/2
  Unit Delay/1 -> Logical Operator2/1
  Logical Operator2/1 -> Logical Operator1/1
  CLEAR/1 -> Unit Delay/1, Logical Operator1/2
  Logical Operator1/1 -> Logical Operator3/1
  MODE/1 -> IS_SETUP/1
  IS_SETUP/1 -> Logical Operator3/2
  Logical Operator3/1 -> implies/1
  Relational Operator/1 -> implies/2
  implies/1 -> OK/1

== system microwave_class_updated/microwave/MODE_CONTROL/MODE_CONTROL_PROPERTIES/ASSUME_SECONDS_TO_COOK_GT_0 ==
  Seconds_To_Cook : Inport
  Constant : Constant  Value=0
  Relational Operator : RelationalOperator  OutDataTypeStr=boolean
  OK : Outport
  wires:
  Seconds_To_Cook/1 -> Relational Operator/1
  Constant/1 -> Relational Operator/2
  Relational Operator/1 -> OK/1

== system microwave_class_updated/microwave/MODE_CONTROL/MODE_CONTROL_PROPERTIES/HEATING_ELEMENT_1 ==
  note: guarantee "heating_element_on implies door_closed_sensor" :
      | 			heating_element_on => door_closed;
  HEATING_ELEMENT_ON : Inport
  DOOR_CLOSED : Inport  Port=2
  implies : microwave_class_defs/implies
  OK : Outport
  wires:
  HEATING_ELEMENT_ON/1 -> implies/1
  implies/1 -> OK/1
  DOOR_CLOSED/1 -> implies/2

== system microwave_class_updated/microwave/MODE_CONTROL/MODE_CONTROL_PROPERTIES/HEATING_ELEMENT_2 ==
  note: guarantee "heating element on implies time to cook decreases" :
      | 			std.While(heating_element_on) => std.DecreaseInt(seconds_to_cook);
  HEATING_ELEMENT_ON : Inport
  SECONDS_TO_COOK : Inport  Port=2
  Relational Operator : RelationalOperator  Operator=<=  OutDataTypeStr=boolean
  Unit Delay : UnitDelay  SampleTime=-1
  implies : microwave_class_defs/implies
  while : microwave_class_defs/while
  OK : Outport
  wires:
  HEATING_ELEMENT_ON/1 -> while/1
  SECONDS_TO_COOK/1 -> Unit Delay/1, Relational Operator/1
  implies/1 -> OK/1
  Unit Delay/1 -> Relational Operator/2
  Relational Operator/1 -> implies/2
  while/1 -> implies/1

== system microwave_class_updated/microwave/MODE_CONTROL/MODE_CONTROL_PROPERTIES/HEATING_ELEMENT_3 ==
  note: guarantee "time to cook = 0 implies heating_element_off" :
      | 			seconds_to_cook = 0 => not (heating_element_on);
  HEATING_ELEMENT_ON : Inport
  SECONDS_TO_COOK : Inport  Port=2
  Compare To Zero : simulink/Logic and Bit Operations/Compare To Zero  relop===  OutDataTypeStr=boolean
  Logical Operator : Logic  Operator=NOT  AllPortsSameDT=off  OutDataTypeStr=boolean
  implies : microwave_class_defs/implies
  OK : Outport
  wires:
  SECONDS_TO_COOK/1 -> Compare To Zero/1
  HEATING_ELEMENT_ON/1 -> Logical Operator/1
  Compare To Zero/1 -> implies/1
  Logical Operator/1 -> implies/2
  implies/1 -> OK/1

== system microwave_class_updated/microwave/MODE_CONTROL/MODE_CONTROL_PROPERTIES/PROP_CLEAR_TURNS_OFF_COOKING ==
  CLEAR : Inport
  MODE : Inport  Port=2
  IS_COOKING : microwave_class_defs/IS_COOKING
  Logical Operator : Logic  AllPortsSameDT=off  OutDataTypeStr=boolean
  Logical Operator1 : Logic  Operator=NOT  AllPortsSameDT=off  OutDataTypeStr=boolean
  Unit Delay : UnitDelay  SampleTime=-1
  implies : microwave_class_defs/implies
  true_after_first_step : microwave_class_defs/true_after_first_step
  OK : Outport
  wires:
  MODE/1 -> IS_COOKING/1
  IS_COOKING/1 -> Unit Delay/1, Logical Operator1/1
  Logical Operator/1 -> implies/1
  Logical Operator1/1 -> implies/2
  Unit Delay/1 -> Logical Operator/2
  CLEAR/1 -> Logical Operator/1
  implies/1 -> true_after_first_step/1
  true_after_first_step/1 -> OK/1

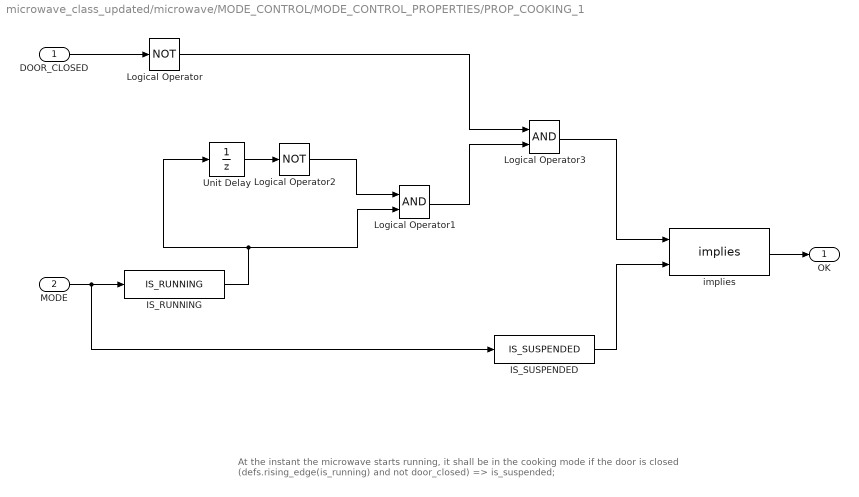
== system microwave_class_updated/microwave/MODE_CONTROL/MODE_CONTROL_PROPERTIES/PROP_COOKING_1 ==
  note: At the instant the microwave starts running, it shall be in the cooking mode if the door is closed
      | (defs.rising_edge(is_running) and not door_closed) => is_suspended;
  DOOR_CLOSED : Inport
  MODE : Inport  Port=2
  IS_RUNNING : microwave_class_defs/IS_RUNNING
  IS_SUSPENDED : microwave_class_defs/IS_SUSPENDED
  Logical Operator : Logic  Operator=NOT  AllPortsSameDT=off  OutDataTypeStr=boolean
  Logical Operator1 : Logic  AllPortsSameDT=off  OutDataTypeStr=boolean
  Logical Operator2 : Logic  Operator=NOT  AllPortsSameDT=off  OutDataTypeStr=boolean
  Logical Operator3 : Logic  AllPortsSameDT=off  OutDataTypeStr=boolean
  Unit Delay : UnitDelay  SampleTime=-1
  implies : microwave_class_defs/implies
  OK : Outport
  wires:
  DOOR_CLOSED/1 -> Logical Operator/1
  Logical Operator/1 -> Logical Operator3/1
  Logical Operator3/1 -> implies/1
  IS_SUSPENDED/1 -> implies/2
  implies/1 -> OK/1
  MODE/1 -> IS_SUSPENDED/1, IS_RUNNING/1
  IS_RUNNING/1 -> Logical Operator1/2, Unit Delay/1
  Unit Delay/1 -> Logical Operator2/1
  Logical Operator2/1 -> Logical Operator1/1
  Logical Operator1/1 -> Logical Operator3/2

== system microwave_class_updated/microwave/MODE_CONTROL/MODE_CONTROL_PROPERTIES/PROP_COOKING_IMPLIES_DOOR_CLOSED ==
  DOOR_CLOSED : Inport
  MODE : Inport  Port=2
  IS_COOKING : microwave_class_defs/IS_COOKING
  implies : Subsystem
  Out1 : Outport
  wires:
  implies/1(A_IMPLIES_B) -> Out1/1
  MODE/1 -> IS_COOKING/1
  DOOR_CLOSED/1 -> implies/2(B)
  IS_COOKING/1 -> implies/1(A)

== system microwave_class_updated/microwave/MODE_CONTROL/MODE_CONTROL_PROPERTIES/PROP_INITIAL_MODE_SETUP ==
  note: The microwave shall be in setup mode in the initial state.
      | std.Initially(is_setup);
  MODE : Inport
  IS_SETUP : microwave_class_defs/IS_SETUP
  initially_true : microwave_class_defs/initially_true
  OK : Outport
  wires:
  initially_true/1 -> OK/1
  MODE/1 -> IS_SETUP/1
  IS_SETUP/1 -> initially_true/1

== system microwave_class_updated/microwave/MODE_CONTROL/MODE_CONTROL_PROPERTIES/PROP_MODE_RANGE ==
  MODE : Inport
  Constant : Constant
  Constant1 : Constant  Value=2
  Constant2 : Constant  Value=3
  Logical Operator : Logic  Operator=OR  Inputs=3  AllPortsSameDT=off  OutDataTypeStr=boolean
  Relational Operator : RelationalOperator  Operator===  OutDataTypeStr=boolean
  Relational Operator1 : RelationalOperator  Operator===  OutDataTypeStr=boolean
  Relational Operator2 : RelationalOperator  Operator===  OutDataTypeStr=boolean
  OK : Outport
  wires:
  Constant/1 -> Relational Operator/2
  Constant1/1 -> Relational Operator1/2
  Constant2/1 -> Relational Operator2/2
  MODE/1 -> Relational Operator2/1, Relational Operator1/1, Relational Operator/1
  Relational Operator/1 -> Logical Operator/1
  Relational Operator1/1 -> Logical Operator/2
  Relational Operator2/1 -> Logical Operator/3
  Logical Operator/1 -> OK/1

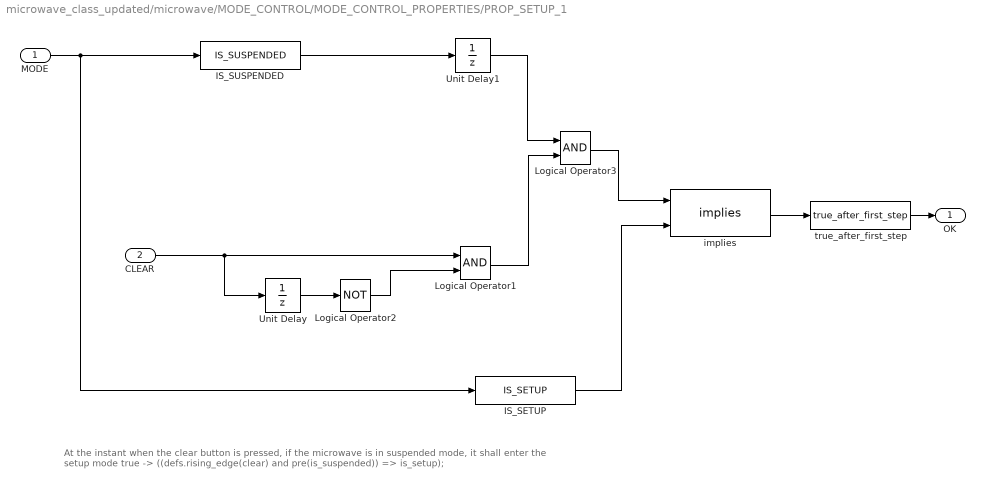
== system microwave_class_updated/microwave/MODE_CONTROL/MODE_CONTROL_PROPERTIES/PROP_SETUP_1 ==
  note: At the instant when the clear button is pressed, if the microwave is in suspended mode, it shall enter the setup mode
      | true ->  ((defs.rising_edge(clear) and pre(is_suspended)) => is_setup);
  MODE : Inport
  CLEAR : Inport  Port=2
  IS_SETUP : microwave_class_defs/IS_SETUP
  IS_SUSPENDED : microwave_class_defs/IS_SUSPENDED
  Logical Operator1 : Logic  AllPortsSameDT=off  OutDataTypeStr=boolean
  Logical Operator2 : Logic  Operator=NOT  AllPortsSameDT=off  OutDataTypeStr=boolean
  Logical Operator3 : Logic  AllPortsSameDT=off  OutDataTypeStr=boolean
  Unit Delay : UnitDelay  SampleTime=-1
  Unit Delay1 : UnitDelay  SampleTime=-1
  implies : microwave_class_defs/implies
  true_after_first_step : microwave_class_defs/true_after_first_step
  OK : Outport
  wires:
  CLEAR/1 -> Unit Delay/1, Logical Operator1/1
  Unit Delay/1 -> Logical Operator2/1
  Logical Operator2/1 -> Logical Operator1/2
  true_after_first_step/1 -> OK/1
  MODE/1 -> IS_SUSPENDED/1, IS_SETUP/1
  IS_SUSPENDED/1 -> Unit Delay1/1
  Unit Delay1/1 -> Logical Operator3/1
  Logical Operator1/1 -> Logical Operator3/2
  Logical Operator3/1 -> implies/1
  IS_SETUP/1 -> implies/2
  implies/1 -> true_after_first_step/1

== system microwave_class_updated/microwave/MODE_CONTROL/MODE_CONTROL_PROPERTIES/PROP_SETUP_2 ==
  note: If seconds_to_cook = 0, microwave will be in setup mode
      | (seconds_to_cook = 0) => is_setup;
  SECONDS_TO_COOK : Inport
  MODE : Inport  Port=2
  Compare To Zero : simulink/Logic and Bit Operations/Compare To Zero  relop===  OutDataTypeStr=boolean
  IS_SETUP : microwave_class_defs/IS_SETUP
  implies : microwave_class_defs/implies
  OK : Outport
  wires:
  SECONDS_TO_COOK/1 -> Compare To Zero/1
  MODE/1 -> IS_SETUP/1
  Compare To Zero/1 -> implies/1
  IS_SETUP/1 -> implies/2
  implies/1 -> OK/1

== system microwave_class_updated/microwave/MODE_CONTROL/MODE_CONTROL_PROPERTIES/PROP_SUSPENDED_1 ==
  note: At the instant the microwave starts running, it shall enter the suspended mode if the door is open
      | (defs.rising_edge(is_running) and not door_closed) => is_suspended;
  MODE : Inport
  DOOR_CLOSED : Inport  Port=2
  IS_RUNNING : microwave_class_defs/IS_RUNNING
  IS_SUSPENDED : microwave_class_defs/IS_SUSPENDED
  Logical Operator : Logic  Operator=NOT  AllPortsSameDT=off  OutDataTypeStr=boolean
  Logical Operator1 : Logic  AllPortsSameDT=off  OutDataTypeStr=boolean
  implies : microwave_class_defs/implies
  OK : Outport
  wires:
  MODE/1 -> IS_SUSPENDED/1, IS_RUNNING/1
  DOOR_CLOSED/1 -> Logical Operator/1
  Logical Operator/1 -> Logical Operator1/2
  IS_RUNNING/1 -> Logical Operator1/1
  implies/1 -> OK/1
  Logical Operator1/1 -> implies/1
  IS_SUSPENDED/1 -> implies/2

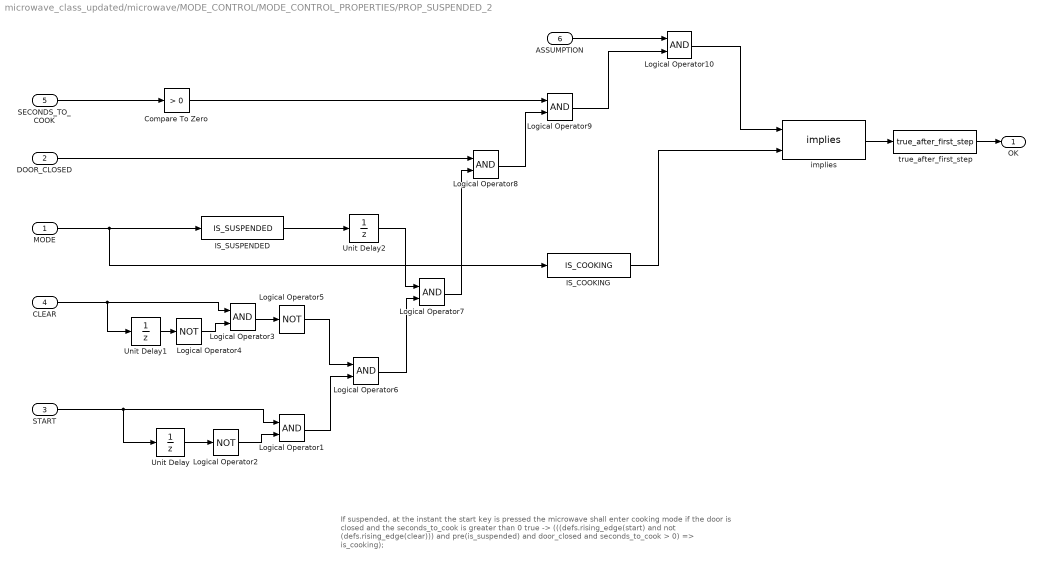
== system microwave_class_updated/microwave/MODE_CONTROL/MODE_CONTROL_PROPERTIES/PROP_SUSPENDED_2 ==
  note: If suspended, at the instant the start key is pressed the microwave shall enter cooking mode if the door is closed and the seconds_to_cook is greater than 0
      | true ->
      | 				(((defs.rising_edge(start) and not (defs.rising_edge(clear))) and
      | 					pre(is_suspended) and door_closed and
      | 					seconds_to_cook > 0) => is_cooking);
  MODE : Inport
  DOOR_CLOSED : Inport  Port=2
  START : Inport  Port=3
  CLEAR : Inport  Port=4
  SECONDS_TO_COOK : Inport  Port=5
  ASSUMPTION : Inport  Port=6
  Compare To Zero : simulink/Logic and Bit Operations/Compare To Zero  relop=>  OutDataTypeStr=boolean
  IS_COOKING : microwave_class_defs/IS_COOKING
  IS_SUSPENDED : microwave_class_defs/IS_SUSPENDED
  Logical Operator{1,3,6..10} (7 alike) : Logic  AllPortsSameDT=off  OutDataTypeStr=boolean
  Logical Operator2 : Logic  Operator=NOT  AllPortsSameDT=off  OutDataTypeStr=boolean
  Logical Operator4 : Logic  Operator=NOT  AllPortsSameDT=off  OutDataTypeStr=boolean
  Logical Operator5 : Logic  Operator=NOT  AllPortsSameDT=off  OutDataTypeStr=boolean
  Unit Delay : UnitDelay  SampleTime=-1
  Unit Delay1 : UnitDelay  SampleTime=-1
  Unit Delay2 : UnitDelay  SampleTime=-1
  implies : microwave_class_defs/implies
  true_after_first_step : microwave_class_defs/true_after_first_step
  OK : Outport
  wires:
  true_after_first_step/1 -> OK/1
  implies/1 -> true_after_first_step/1
  Unit Delay/1 -> Logical Operator2/1
  Logical Operator2/1 -> Logical Operator1/2
  START/1 -> Unit Delay/1, Logical Operator1/1
  Unit Delay1/1 -> Logical Operator4/1
  Logical Operator4/1 -> Logical Operator3/2
  CLEAR/1 -> Unit Delay1/1, Logical Operator3/1
  Logical Operator3/1 -> Logical Operator5/1
  Logical Operator5/1 -> Logical Operator6/1
  Logical Operator1/1 -> Logical Operator6/2
  MODE/1 -> IS_COOKING/1, IS_SUSPENDED/1
  IS_SUSPENDED/1 -> Unit Delay2/1
  Unit Delay2/1 -> Logical Operator7/1
  Logical Operator6/1 -> Logical Operator7/2
  DOOR_CLOSED/1 -> Logical Operator8/1
  Logical Operator7/1 -> Logical Operator8/2
  SECONDS_TO_COOK/1 -> Compare To Zero/1
  Compare To Zero/1 -> Logical Operator9/1
  Logical Operator8/1 -> Logical Operator9/2
  Logical Operator9/1 -> Logical Operator10/2
  IS_COOKING/1 -> implies/2
  ASSUMPTION/1 -> Logical Operator10/1
  Logical Operator10/1 -> implies/1

== system microwave_class_updated/microwave/MODE_CONTROL/MODE_CONTROL_PROPERTIES/PROP_COOKING_IMPLIES_DOOR_CLOSED/implies ==
  A : Inport
  B : Inport  Port=2
  Logical Operator : Logic  Operator=OR  AllPortsSameDT=off  OutDataTypeStr=boolean
  Logical Operator1 : Logic  Operator=NOT  AllPortsSameDT=off  OutDataTypeStr=boolean
  A_IMPLIES_B : Outport
  wires:
  A/1 -> Logical Operator1/1
  B/1 -> Logical Operator/2
  Logical Operator1/1 -> Logical Operator/1
  Logical Operator/1 -> A_IMPLIES_B/1

== stateflow chart microwave/MODE_CONTROL/MODE_CONTROL ==
  state SUSPENDED
    en, du:
    HEATING_ELEMENT_ON = false;
  state COOKING
    en, du:
    HEATING_ELEMENT_ON = true;
  state SETUP
    en, du:
    HEATING_ELEMENT_ON = false;
  COOKING -> SETUP [order 1] : [SECONDS_TO_COOK == 0] {COOKING_MODE = 1;}
  COOKING -> COOKING [order 2] : [KP_START]
  (default) -> SETUP : {COOKING_MODE = 1;}
  SETUP -> COOKING [order 1] : [KP_START && SECONDS_TO_COOK > 0  && DOOR_CLOSED] {COOKING_MODE = 3;}
  SUSPENDED -> SETUP [order 1] : [SECONDS_TO_COOK == 0 || KP_CLEAR] {COOKING_MODE = 1;}
  SETUP -> SUSPENDED [order 2] : [KP_START && SECONDS_TO_COOK > 0 && ~DOOR_CLOSED] {COOKING_MODE = 2;}
  SUSPENDED -> COOKING [order 2] : [DOOR_CLOSED && KP_START && SECONDS_TO_COOK > 0] {COOKING_MODE = 3;}
  COOKING -> SUSPENDED [order 3] : [KP_CLEAR ||  ~DOOR_CLOSED] {COOKING_MODE = 2;}
  data: KP_START input boolean; KP_CLEAR input boolean; DOOR_CLOSED input boolean; SECONDS_TO_COOK input int8; COOKING_MODE output uint8; HEATING_ELEMENT_ON output boolean

== stateflow chart microwave/DISPLAY_CONTROL/DISPLAY_CONTROL ==
  state SETUP
    en:
    LEFT_DIGIT = int8(0);
    RIGHT_DIGIT = int8(0);
    MIDDLE_DIGIT = int8(0);
    en, ex:
    SECONDS_TO_COOK = 0;
  state SUSPENDED
    en, du, ex:
    SECONDS_TO_COOK = LEFT_DIGIT * 60 +  MIDDLE_DIGIT * 10 +  RIGHT_DIGIT;
  state COOKING
    en, du, ex:
    SECONDS_TO_COOK = LEFT_DIGIT * 60 +  MIDDLE_DIGIT * 10 +  RIGHT_DIGIT;
    du:
    SECONDS_TO_COOK = SECONDS_TO_COOK - STEP;
    LEFT_DIGIT =  SECONDS_TO_COOK / 60;
    MIDDLE_DIGIT = (SECONDS_TO_COOK %%   60)/ 10;
    RIGHT_DIGIT = (SECONDS_TO_COOK %%  60) %% 10;
  state RIGHT_DG
    en, ex:
    SECONDS_TO_COOK = LEFT_DIGIT * 60 +  MIDDLE_DIGIT * 10 +  RIGHT_DIGIT;
  state LEFT_DG
    en, ex:
    SECONDS_TO_COOK = LEFT_DIGIT * 60 +  MIDDLE_DIGIT * 10 +  RIGHT_DIGIT;
  state MID_DG
    en, ex:
    SECONDS_TO_COOK = LEFT_DIGIT * 60 +  MIDDLE_DIGIT * 10 +  RIGHT_DIGIT;
  note: [KP_CLEAR]
  note: [COOKING_MODE == 3]
  SUSPENDED -> SETUP [order 1] : [COOKING_MODE == 1]
  COOKING -> SUSPENDED [order 1] : [COOKING_MODE == 2]
  SUSPENDED -> COOKING [order 2] : [COOKING_MODE == 3]
  SETUP -> SETUP [order 1] : [KP_CLEAR]
  (default) -> SETUP
  (junction 38) -> SETUP
  COOKING -> SETUP [order 2] : [SECONDS_TO_COOK == 0]
  SETUP -> RIGHT_DG [order 2] : [DIGIT_PRESSED >= 0 && COOKING_MODE == 1] {RIGHT_DIGIT = DIGIT_PRESSED; }
  (junction 39) -> COOKING
  RIGHT_DG -> (junction 38) [order 1]
  RIGHT_DG -> (junction 39) [order 2]
  RIGHT_DG -> MID_DG [order 3] : [DIGIT_PRESSED >= 0 && COOKING_MODE == 1] {MIDDLE_DIGIT = RIGHT_DIGIT; RIGHT_DIGIT = DIGIT_PRESSED;}
  MID_DG -> (junction 38) [order 1]
  MID_DG -> (junction 39) [order 2]
  LEFT_DG -> (junction 38) [order 1]
  LEFT_DG -> (junction 39) [order 2]
  MID_DG -> LEFT_DG [order 3] : [DIGIT_PRESSED >= 0 && COOKING_MODE == 1] {LEFT_DIGIT = MIDDLE_DIGIT; MIDDLE_DIGIT = RIGHT_DIGIT; RIGHT_DIGIT = DIGIT_PRESSED;}
  LEFT_DG -> LEFT_DG [order 3] : [DIGIT_PRESSED >=  0]
  data: LEFT_DIGIT output int8; MIDDLE_DIGIT output int8; RIGHT_DIGIT output int8; STEP input int8; KP_CLEAR input double; DIGIT_PRESSED input int8; SECONDS_TO_COOK output int8; COOKING_MODE input double
